simulink library "halin"  (R2021b)
settings: Solver=VariableStepAuto  StartTime=0.0  StopTime=10.0  RelTol=1e-3
undefined symbols (not defined in the file): TRUE
libraries: FVT_lib x177, hcu_lib x55
(part 16 of 17)

== system halin/HAL_IN/CAN4/ZONE_DR_VCU/TFootRErr ==
  T_Foot_R_Err : Inport
  UnitConverter : DataTypeConversion  OutDataTypeStr=uint8
  VHAL_TFootRErr_enum : Outport
  wires:
  UnitConverter/1 -> VHAL_TFootRErr_enum/1
  T_Foot_R_Err/1 -> UnitConverter/1

== system halin/HAL_IN/CAN4/ZONE_DR_VCU/TFootRr ==
  T_Foot_Rr : Inport
  UnitConverter : DataTypeConversion  OutDataTypeStr=uint8
  convert_in : FVT_lib/hal/convert_in  gain=0.5  offset=-40
  VHAL_TFootRr_C : Outport
  wires:
  convert_in/1 -> VHAL_TFootRr_C/1
  UnitConverter/1 -> convert_in/1
  T_Foot_Rr/1 -> UnitConverter/1

== system halin/HAL_IN/CAN4/ZONE_DR_VCU/TFootRrErr ==
  T_Foot_Rr_Err : Inport
  UnitConverter : DataTypeConversion  OutDataTypeStr=uint8
  VHAL_TFootRrErr_enum : Outport
  wires:
  UnitConverter/1 -> VHAL_TFootRrErr_enum/1
  T_Foot_Rr_Err/1 -> UnitConverter/1

== system halin/HAL_IN/CAN4/ZONE_DR_VCU/Tevap ==
  Tevap : Inport
  UnitConverter : DataTypeConversion  OutDataTypeStr=uint8
  convert_in : FVT_lib/hal/convert_in  gain=0.5  offset=-40
  VHAL_Tevap_C : Outport
  wires:
  convert_in/1 -> VHAL_Tevap_C/1
  UnitConverter/1 -> convert_in/1
  Tevap/1 -> UnitConverter/1

== system halin/HAL_IN/CAN4/ZONE_DR_VCU/TevapErr ==
  Tevap_Err : Inport
  UnitConverter : DataTypeConversion  OutDataTypeStr=uint8
  VHAL_TevapErr_enum : Outport
  wires:
  UnitConverter/1 -> VHAL_TevapErr_enum/1
  Tevap_Err/1 -> UnitConverter/1

== system halin/HAL_IN/CAN4/ZONE_DR_VCU/Tincar ==
  Tincar : Inport
  UnitConverter : DataTypeConversion  OutDataTypeStr=uint8
  convert_in : FVT_lib/hal/convert_in  gain=0.5  offset=-40
  VHAL_Tincar_C : Outport
  wires:
  convert_in/1 -> VHAL_Tincar_C/1
  UnitConverter/1 -> convert_in/1
  Tincar/1 -> UnitConverter/1

== system halin/HAL_IN/CAN4/ZONE_DR_VCU/TincarErr ==
  Tincar_Err : Inport
  UnitConverter : DataTypeConversion  OutDataTypeStr=uint8
  VHAL_TincarErr_enum : Outport
  wires:
  UnitConverter/1 -> VHAL_TincarErr_enum/1
  Tincar_Err/1 -> UnitConverter/1

== system halin/HAL_IN/CAN4/ZONE_DR_VCU/ZoneDrMalfunLevel ==
  ZoneDrMalfunLevel : Inport
  UnitConverter : DataTypeConversion  OutDataTypeStr=uint8
  VHAL_ZoneDrMalfunLevel_enum : Outport
  wires:
  UnitConverter/1 -> VHAL_ZoneDrMalfunLevel_enum/1
  ZoneDrMalfunLevel/1 -> UnitConverter/1

== system halin/HAL_IN/CAN4/ZONE_FR1/ChargeInletLockSta ==
  ChargeInletLockSta : Inport
  UnitConverter : DataTypeConversion  OutDataTypeStr=uint8
  VHAL_ChargeInletLockSta_flg : Outport
  wires:
  UnitConverter/1 -> VHAL_ChargeInletLockSta_flg/1
  ChargeInletLockSta/1 -> UnitConverter/1

== system halin/HAL_IN/CAN4/ZONE_FR1/CompProEN ==
  CompProEN : Inport
  UnitConverter : DataTypeConversion  OutDataTypeStr=uint8
  VHAL_CompProEN_flg : Outport
  wires:
  UnitConverter/1 -> VHAL_CompProEN_flg/1
  CompProEN/1 -> UnitConverter/1

== system halin/HAL_IN/CAN4/ZONE_FR1/FLTurnLampC ==
  FLTurnLampC : Inport
  UnitConverter : DataTypeConversion  OutDataTypeStr=uint8
  convert_in : FVT_lib/hal/convert_in  gain=10  offset=0
  VHAL_FLTurnLampC_mA : Outport
  wires:
  convert_in/1 -> VHAL_FLTurnLampC_mA/1
  UnitConverter/1 -> convert_in/1
  FLTurnLampC/1 -> UnitConverter/1

== system halin/HAL_IN/CAN4/ZONE_FR1/FLTurnLightWarning ==
  FLTurn_Light_Warning : Inport
  UnitConverter : DataTypeConversion  OutDataTypeStr=uint8
  VHAL_FLTurnLightWarning_flg : Outport
  wires:
  UnitConverter/1 -> VHAL_FLTurnLightWarning_flg/1
  FLTurn_Light_Warning/1 -> UnitConverter/1

== system halin/HAL_IN/CAN4/ZONE_FR1/FRTurnLampC ==
  FRTurnLampC : Inport
  UnitConverter : DataTypeConversion  OutDataTypeStr=uint8
  convert_in : FVT_lib/hal/convert_in  gain=10  offset=0
  VHAL_FRTurnLampC_mA : Outport
  wires:
  convert_in/1 -> VHAL_FRTurnLampC_mA/1
  UnitConverter/1 -> convert_in/1
  FRTurnLampC/1 -> UnitConverter/1

== system halin/HAL_IN/CAN4/ZONE_FR1/FRTurnLightWarning ==
  FRTurn_Light_Warning : Inport
  UnitConverter : DataTypeConversion  OutDataTypeStr=uint8
  VHAL_FRTurnLightWarning_flg : Outport
  wires:
  UnitConverter/1 -> VHAL_FRTurnLightWarning_flg/1
  FRTurn_Light_Warning/1 -> UnitConverter/1

== system halin/HAL_IN/CAN4/ZONE_FR1/FWiperAS ==
  FWiperAS : Inport
  UnitConverter : DataTypeConversion  OutDataTypeStr=uint8
  VHAL_FWiperAS_flg : Outport
  wires:
  UnitConverter/1 -> VHAL_FWiperAS_flg/1
  FWiperAS/1 -> UnitConverter/1

== system halin/HAL_IN/CAN4/ZONE_FR1/FWiperProtection ==
  FWiperProtection : Inport
  UnitConverter : DataTypeConversion  OutDataTypeStr=uint8
  VHAL_FWiperProtection_flg : Outport
  wires:
  UnitConverter/1 -> VHAL_FWiperProtection_flg/1
  FWiperProtection/1 -> UnitConverter/1

== system halin/HAL_IN/CAN4/ZONE_FR1/LADBHibeamIndication ==
  LADB_Hibeam_Indication : Inport
  UnitConverter : DataTypeConversion  OutDataTypeStr=uint8
  VHAL_LADBHibeamIndication_flg : Outport
  wires:
  UnitConverter/1 -> VHAL_LADBHibeamIndication_flg/1
  LADB_Hibeam_Indication/1 -> UnitConverter/1

== system halin/HAL_IN/CAN4/ZONE_FR1/LADBOperationStatus ==
  LADB_Operation_Status : Inport
  UnitConverter : DataTypeConversion  OutDataTypeStr=uint8
  VHAL_LADBOperationStatus_flg : Outport
  wires:
  UnitConverter/1 -> VHAL_LADBOperationStatus_flg/1
  LADB_Operation_Status/1 -> UnitConverter/1

== system halin/HAL_IN/CAN4/ZONE_FR1/LADBWarning ==
  LADB_Warning : Inport
  UnitConverter : DataTypeConversion  OutDataTypeStr=uint8
  VHAL_LADBWarning_flg : Outport
  wires:
  UnitConverter/1 -> VHAL_LADBWarning_flg/1
  LADB_Warning/1 -> UnitConverter/1

== system halin/HAL_IN/CAN4/ZONE_FR1/LAHBWarning ==
  LAHB_Warning : Inport
  UnitConverter : DataTypeConversion  OutDataTypeStr=uint8
  VHAL_LAHBWarning_flg : Outport
  wires:
  UnitConverter/1 -> VHAL_LAHBWarning_flg/1
  LAHB_Warning/1 -> UnitConverter/1

== system halin/HAL_IN/CAN4/ZONE_FR1/LDRLWarning ==
  LDRL_Warning : Inport
  UnitConverter : DataTypeConversion  OutDataTypeStr=uint8
  VHAL_LDRLWarning_flg : Outport
  wires:
  UnitConverter/1 -> VHAL_LDRLWarning_flg/1
  LDRL_Warning/1 -> UnitConverter/1

== system halin/HAL_IN/CAN4/ZONE_FR1/LLBWarning ==
  LLB_Warning : Inport
  UnitConverter : DataTypeConversion  OutDataTypeStr=uint8
  VHAL_LLBWarning_flg : Outport
  wires:
  UnitConverter/1 -> VHAL_LLBWarning_flg/1
  LLB_Warning/1 -> UnitConverter/1

== system halin/HAL_IN/CAN4/ZONE_FR1/LpositionLampWarning ==
  Lposition_Lamp_Warning : Inport
  UnitConverter : DataTypeConversion  OutDataTypeStr=uint8
  VHAL_LpositionLampWarning_flg : Outport
  wires:
  UnitConverter/1 -> VHAL_LpositionLampWarning_flg/1
  Lposition_Lamp_Warning/1 -> UnitConverter/1

== system halin/HAL_IN/CAN4/ZONE_FR1/RADBHibeamIndication ==
  RADB_Hibeam_Indication : Inport
  UnitConverter : DataTypeConversion  OutDataTypeStr=uint8
  VHAL_RADBHibeamIndication_flg : Outport
  wires:
  UnitConverter/1 -> VHAL_RADBHibeamIndication_flg/1
  RADB_Hibeam_Indication/1 -> UnitConverter/1

== system halin/HAL_IN/CAN4/ZONE_FR1/RADBOperationStatus ==
  RADB_Operation_Status : Inport
  UnitConverter : DataTypeConversion  OutDataTypeStr=uint8
  VHAL_RADBOperationStatus_flg : Outport
  wires:
  UnitConverter/1 -> VHAL_RADBOperationStatus_flg/1
  RADB_Operation_Status/1 -> UnitConverter/1

== system halin/HAL_IN/CAN4/ZONE_FR1/RADBWarning ==
  RADB_Warning : Inport
  UnitConverter : DataTypeConversion  OutDataTypeStr=uint8
  VHAL_RADBWarning_flg : Outport
  wires:
  UnitConverter/1 -> VHAL_RADBWarning_flg/1
  RADB_Warning/1 -> UnitConverter/1

== system halin/HAL_IN/CAN4/ZONE_FR1/RAHBWarning ==
  RAHB_Warning : Inport
  UnitConverter : DataTypeConversion  OutDataTypeStr=uint8
  VHAL_RAHBWarning_flg : Outport
  wires:
  UnitConverter/1 -> VHAL_RAHBWarning_flg/1
  RAHB_Warning/1 -> UnitConverter/1

== system halin/HAL_IN/CAN4/ZONE_FR1/RDRLWarning ==
  RDRL_Warning : Inport
  UnitConverter : DataTypeConversion  OutDataTypeStr=uint8
  VHAL_RDRLWarning_flg : Outport
  wires:
  UnitConverter/1 -> VHAL_RDRLWarning_flg/1
  RDRL_Warning/1 -> UnitConverter/1

== system halin/HAL_IN/CAN4/ZONE_FR1/RLBWarning ==
  RLB_Warning : Inport
  UnitConverter : DataTypeConversion  OutDataTypeStr=uint8
  VHAL_RLBWarning_flg : Outport
  wires:
  UnitConverter/1 -> VHAL_RLBWarning_flg/1
  RLB_Warning/1 -> UnitConverter/1

== system halin/HAL_IN/CAN4/ZONE_FR1/RpositionLampWarning ==
  Rposition_Lamp_Warning : Inport
  UnitConverter : DataTypeConversion  OutDataTypeStr=uint8
  VHAL_RpositionLampWarning_flg : Outport
  wires:
  UnitConverter/1 -> VHAL_RpositionLampWarning_flg/1
  Rposition_Lamp_Warning/1 -> UnitConverter/1

== system halin/HAL_IN/CAN4/ZONE_FR1/TrailerCheck ==
  TrailerCheck : Inport
  UnitConverter : DataTypeConversion  OutDataTypeStr=uint8
  VHAL_TrailerCheck_flg : Outport
  wires:
  UnitConverter/1 -> VHAL_TrailerCheck_flg/1
  TrailerCheck/1 -> UnitConverter/1

== system halin/HAL_IN/CAN4/ZONE_FR1/TrailerModeSta ==
  TrailerModeSta : Inport
  UnitConverter : DataTypeConversion  OutDataTypeStr=uint8
  VHAL_TrailerModeSta_enum : Outport
  wires:
  UnitConverter/1 -> VHAL_TrailerModeSta_enum/1
  TrailerModeSta/1 -> UnitConverter/1

== system halin/HAL_IN/CAN4/ZONE_FR1/ZFRBCMChargerDoorSWSta ==
  ZFR_BCM_ChargerDoorSW_Sta : Inport
  UnitConverter : DataTypeConversion  OutDataTypeStr=uint8
  VHAL_ZFRBCMChargerDoorSWSta_flg : Outport
  wires:
  UnitConverter/1 -> VHAL_ZFRBCMChargerDoorSWSta_flg/1
  ZFR_BCM_ChargerDoorSW_Sta/1 -> UnitConverter/1

== system halin/HAL_IN/CAN4/ZONE_FR1/ZFRTHCMCLEVentActYSta ==
  ZFR_THCM_CLEVentActY_Sta : Inport
  UnitConverter : DataTypeConversion  OutDataTypeStr=uint8
  VHAL_ZFRTHCMCLEVentActYSta_pct : Outport
  wires:
  UnitConverter/1 -> VHAL_ZFRTHCMCLEVentActYSta_pct/1
  ZFR_THCM_CLEVentActY_Sta/1 -> UnitConverter/1

== system halin/HAL_IN/CAN4/ZONE_FR1/ZFRTHCMCREVentActYSta ==
  ZFR_THCM_CREVentActY_Sta : Inport
  UnitConverter : DataTypeConversion  OutDataTypeStr=uint8
  VHAL_ZFRTHCMCREVentActYSta_pct : Outport
  wires:
  UnitConverter/1 -> VHAL_ZFRTHCMCREVentActYSta_pct/1
  ZFR_THCM_CREVentActY_Sta/1 -> UnitConverter/1

== system halin/HAL_IN/CAN4/ZONE_FR1/ZFRTHCMDrEVentActYSta ==
  ZFR_THCM_DrEVentActY_Sta : Inport
  UnitConverter : DataTypeConversion  OutDataTypeStr=uint8
  VHAL_ZFRTHCMDrEVentActYSta_pct : Outport
  wires:
  UnitConverter/1 -> VHAL_ZFRTHCMDrEVentActYSta_pct/1
  ZFR_THCM_DrEVentActY_Sta/1 -> UnitConverter/1

== system halin/HAL_IN/CAN4/ZONE_FR1/ZFRTHCMPsEVentActYSta ==
  ZFR_THCM_PsEVentActY_Sta : Inport
  UnitConverter : DataTypeConversion  OutDataTypeStr=uint8
  VHAL_ZFRTHCMPsEVentActYSta_pct : Outport
  wires:
  UnitConverter/1 -> VHAL_ZFRTHCMPsEVentActYSta_pct/1
  ZFR_THCM_PsEVentActY_Sta/1 -> UnitConverter/1

== system halin/HAL_IN/CAN4/ZONE_FR_VCU/AGSErr ==
  AGS_Err : Inport
  UnitConverter : DataTypeConversion  OutDataTypeStr=uint8
  VHAL_AGSErr_enum : Outport
  wires:
  UnitConverter/1 -> VHAL_AGSErr_enum/1
  AGS_Err/1 -> UnitConverter/1

== system halin/HAL_IN/CAN4/ZONE_FR_VCU/BatInTemp ==
  Bat_In_Temp : Inport
  UnitConverter : DataTypeConversion  OutDataTypeStr=uint8
  convert_in : FVT_lib/hal/convert_in  gain=0.5  offset=-40
  VHAL_BatInTemp_C : Outport
  wires:
  convert_in/1 -> VHAL_BatInTemp_C/1
  UnitConverter/1 -> convert_in/1
  Bat_In_Temp/1 -> UnitConverter/1

== system halin/HAL_IN/CAN4/ZONE_FR_VCU/BatInTempErr ==
  Bat_In_Temp_Err : Inport
  UnitConverter : DataTypeConversion  OutDataTypeStr=uint8
  VHAL_BatInTempErr_enum : Outport
  wires:
  UnitConverter/1 -> VHAL_BatInTempErr_enum/1
  Bat_In_Temp_Err/1 -> UnitConverter/1

== system halin/HAL_IN/CAN4/ZONE_FR_VCU/BatOutTemp ==
  Bat_Out_Temp : Inport
  UnitConverter : DataTypeConversion  OutDataTypeStr=uint8
  convert_in : FVT_lib/hal/convert_in  gain=0.5  offset=-40
  VHAL_BatOutTemp_C : Outport
  wires:
  convert_in/1 -> VHAL_BatOutTemp_C/1
  UnitConverter/1 -> convert_in/1
  Bat_Out_Temp/1 -> UnitConverter/1

== system halin/HAL_IN/CAN4/ZONE_FR_VCU/COMPErr ==
  COMP_Err : Inport
  UnitConverter : DataTypeConversion  OutDataTypeStr=uint8
  VHAL_COMPErr_enum : Outport
  wires:
  UnitConverter/1 -> VHAL_COMPErr_enum/1
  COMP_Err/1 -> UnitConverter/1

== system halin/HAL_IN/CAN4/ZONE_FR_VCU/EACProtectEnable ==
  EACProtectEnable : Inport
  UnitConverter : DataTypeConversion  OutDataTypeStr=uint8
  VHAL_EACProtectEnable_enum : Outport
  wires:
  UnitConverter/1 -> VHAL_EACProtectEnable_enum/1
  EACProtectEnable/1 -> UnitConverter/1

== system halin/HAL_IN/CAN4/ZONE_FR_VCU/EWP3Err ==
  EWP3_Err : Inport
  UnitConverter : DataTypeConversion  OutDataTypeStr=uint8
  VHAL_EWP3Err_enum : Outport
  wires:
  UnitConverter/1 -> VHAL_EWP3Err_enum/1
  EWP3_Err/1 -> UnitConverter/1

== system halin/HAL_IN/CAN4/ZONE_FR_VCU/EXV1Err ==
  EXV1_Err : Inport
  UnitConverter : DataTypeConversion  OutDataTypeStr=uint8
  VHAL_EXV1Err_enum : Outport
  wires:
  UnitConverter/1 -> VHAL_EXV1Err_enum/1
  EXV1_Err/1 -> UnitConverter/1

== system halin/HAL_IN/CAN4/ZONE_FR_VCU/EXV2Err ==
  EXV2_Err : Inport
  UnitConverter : DataTypeConversion  OutDataTypeStr=uint8
  VHAL_EXV2Err_enum : Outport
  wires:
  UnitConverter/1 -> VHAL_EXV2Err_enum/1
  EXV2_Err/1 -> UnitConverter/1

== system halin/HAL_IN/CAN4/ZONE_FR_VCU/FanErr ==
  Fan_Err : Inport
  UnitConverter : DataTypeConversion  OutDataTypeStr=uint8
  VHAL_FanErr_enum : Outport
  wires:
  UnitConverter/1 -> VHAL_FanErr_enum/1
  Fan_Err/1 -> UnitConverter/1

== system halin/HAL_IN/CAN4/ZONE_FR_VCU/FrPMMLimpHomeActReq ==
  FrPMMLimpHomeActReq : Inport
  UnitConverter : DataTypeConversion  OutDataTypeStr=uint8
  VHAL_FrPMMLimpHomeActReq_flg : Outport
  wires:
  UnitConverter/1 -> VHAL_FrPMMLimpHomeActReq_flg/1
  FrPMMLimpHomeActReq/1 -> UnitConverter/1

== system halin/HAL_IN/CAN4/ZONE_FR_VCU/MotorInTemp ==
  Motor_In_Temp : Inport
  UnitConverter : DataTypeConversion  OutDataTypeStr=uint8
  convert_in : FVT_lib/hal/convert_in  gain=0.5  offset=-40
  VHAL_MotorInTemp_C : Outport
  wires:
  convert_in/1 -> VHAL_MotorInTemp_C/1
  UnitConverter/1 -> convert_in/1
  Motor_In_Temp/1 -> UnitConverter/1

== system halin/HAL_IN/CAN4/ZONE_FR_VCU/MotorInTempErr ==
  Motor_In_Temp_Err : Inport
  UnitConverter : DataTypeConversion  OutDataTypeStr=uint8
  VHAL_MotorInTempErr_enum : Outport
  wires:
  UnitConverter/1 -> VHAL_MotorInTempErr_enum/1
  Motor_In_Temp_Err/1 -> UnitConverter/1

== system halin/HAL_IN/CAN4/ZONE_FR_VCU/MotorOutTemp ==
  Motor_Out_Temp : Inport
  UnitConverter : DataTypeConversion  OutDataTypeStr=uint8
  convert_in : FVT_lib/hal/convert_in  gain=0.5  offset=-40
  VHAL_MotorOutTemp_C : Outport
  wires:
  convert_in/1 -> VHAL_MotorOutTemp_C/1
  UnitConverter/1 -> convert_in/1
  Motor_Out_Temp/1 -> UnitConverter/1

== system halin/HAL_IN/CAN4/ZONE_FR_VCU/MotorOutTempErr ==
  Motor_Out_Temp_Err : Inport
  UnitConverter : DataTypeConversion  OutDataTypeStr=uint8
  VHAL_MotorOutTempErr_enum : Outport
  wires:
  UnitConverter/1 -> VHAL_MotorOutTempErr_enum/1
  Motor_Out_Temp_Err/1 -> UnitConverter/1

== system halin/HAL_IN/CAN4/ZONE_FR_VCU/PTHighP ==
  PT_High_P : Inport
  UnitConverter : DataTypeConversion  OutDataTypeStr=uint16
  VHAL_PTHighP_KPa : Outport
  wires:
  UnitConverter/1 -> VHAL_PTHighP_KPa/1
  PT_High_P/1 -> UnitConverter/1

== system halin/HAL_IN/CAN4/ZONE_FR_VCU/PTHighPErr ==
  PT_High_P_Err : Inport
  UnitConverter : DataTypeConversion  OutDataTypeStr=uint8
  VHAL_PTHighPErr_enum : Outport
  wires:
  UnitConverter/1 -> VHAL_PTHighPErr_enum/1
  PT_High_P_Err/1 -> UnitConverter/1

== system halin/HAL_IN/CAN4/ZONE_FR_VCU/PTHighTact ==
  PT_High_Tact : Inport
  UnitConverter : DataTypeConversion  OutDataTypeStr=uint8
  convert_in : FVT_lib/hal/convert_in  gain=1  offset=-40
  VHAL_PTHighTact_C : Outport
  wires:
  convert_in/1 -> VHAL_PTHighTact_C/1
  UnitConverter/1 -> convert_in/1
  PT_High_Tact/1 -> UnitConverter/1

== system halin/HAL_IN/CAN4/ZONE_FR_VCU/PTHighTactErr ==
  PT_High_Tact_Err : Inport
  UnitConverter : DataTypeConversion  OutDataTypeStr=uint8
  VHAL_PTHighTactErr_enum : Outport
  wires:
  UnitConverter/1 -> VHAL_PTHighTactErr_enum/1
  PT_High_Tact_Err/1 -> UnitConverter/1

== system halin/HAL_IN/CAN4/ZONE_FR_VCU/PTLowP1 ==
  PT_Low_P1 : Inport
  UnitConverter : DataTypeConversion  OutDataTypeStr=uint16
  VHAL_PTLowP1_KPa : Outport
  wires:
  UnitConverter/1 -> VHAL_PTLowP1_KPa/1
  PT_Low_P1/1 -> UnitConverter/1

== system halin/HAL_IN/CAN4/ZONE_FR_VCU/PTLowP1Err ==
  PT_Low_P1_Err : Inport
  UnitConverter : DataTypeConversion  OutDataTypeStr=uint8
  VHAL_PTLowP1Err_enum : Outport
  wires:
  UnitConverter/1 -> VHAL_PTLowP1Err_enum/1
  PT_Low_P1_Err/1 -> UnitConverter/1

== system halin/HAL_IN/CAN4/ZONE_FR_VCU/PTLowP2 ==
  PT_Low_P2 : Inport
  UnitConverter : DataTypeConversion  OutDataTypeStr=uint16
  VHAL_PTLowP2_KPa : Outport
  wires:
  UnitConverter/1 -> VHAL_PTLowP2_KPa/1
  PT_Low_P2/1 -> UnitConverter/1

== system halin/HAL_IN/CAN4/ZONE_FR_VCU/PTLowP2Err ==
  PT_Low_P2_Err : Inport
  UnitConverter : DataTypeConversion  OutDataTypeStr=uint8
  VHAL_PTLowP2Err_enum : Outport
  wires:
  UnitConverter/1 -> VHAL_PTLowP2Err_enum/1
  PT_Low_P2_Err/1 -> UnitConverter/1

== system halin/HAL_IN/CAN4/ZONE_FR_VCU/PTLowT1 ==
  PT_Low_T1 : Inport
  UnitConverter : DataTypeConversion  OutDataTypeStr=uint8
  convert_in : FVT_lib/hal/convert_in  gain=0.5  offset=-40
  VHAL_PTLowT1_C : Outport
  wires:
  convert_in/1 -> VHAL_PTLowT1_C/1
  UnitConverter/1 -> convert_in/1
  PT_Low_T1/1 -> UnitConverter/1

== system halin/HAL_IN/CAN4/ZONE_FR_VCU/PTLowT1Err ==
  PT_Low_T1_Err : Inport
  UnitConverter : DataTypeConversion  OutDataTypeStr=uint8
  VHAL_PTLowT1Err_enum : Outport
  wires:
  UnitConverter/1 -> VHAL_PTLowT1Err_enum/1
  PT_Low_T1_Err/1 -> UnitConverter/1

== system halin/HAL_IN/CAN4/ZONE_FR_VCU/PTLowT2 ==
  PT_Low_T2 : Inport
  UnitConverter : DataTypeConversion  OutDataTypeStr=uint8
  convert_in : FVT_lib/hal/convert_in  gain=0.5  offset=-40
  VHAL_PTLowT2_C : Outport
  wires:
  convert_in/1 -> VHAL_PTLowT2_C/1
  UnitConverter/1 -> convert_in/1
  PT_Low_T2/1 -> UnitConverter/1

== system halin/HAL_IN/CAN4/ZONE_FR_VCU/PTLowT2Err ==
  PT_Low_T2_Err : Inport
  UnitConverter : DataTypeConversion  OutDataTypeStr=uint8
  VHAL_PTLowT2Err_enum : Outport
  wires:
  UnitConverter/1 -> VHAL_PTLowT2Err_enum/1
  PT_Low_T2_Err/1 -> UnitConverter/1

== system halin/HAL_IN/CAN4/ZONE_FR_VCU/SOTXVErr ==
  SOTXV_Err : Inport
  UnitConverter : DataTypeConversion  OutDataTypeStr=uint8
  VHAL_SOTXVErr_enum : Outport
  wires:
  UnitConverter/1 -> VHAL_SOTXVErr_enum/1
  SOTXV_Err/1 -> UnitConverter/1

== system halin/HAL_IN/CAN4/ZONE_FR_VCU/SOV1Err ==
  SOV1_Err : Inport
  UnitConverter : DataTypeConversion  OutDataTypeStr=uint8
  VHAL_SOV1Err_enum : Outport
  wires:
  UnitConverter/1 -> VHAL_SOV1Err_enum/1
  SOV1_Err/1 -> UnitConverter/1

== system halin/HAL_IN/CAN4/ZONE_FR_VCU/SOV2Err ==
  SOV2_Err : Inport
  UnitConverter : DataTypeConversion  OutDataTypeStr=uint8
  VHAL_SOV2Err_enum : Outport
  wires:
  UnitConverter/1 -> VHAL_SOV2Err_enum/1
  SOV2_Err/1 -> UnitConverter/1

== system halin/HAL_IN/CAN4/ZONE_FR_VCU/SOV3Err ==
  SOV3_Err : Inport
  UnitConverter : DataTypeConversion  OutDataTypeStr=uint8
  VHAL_SOV3Err_enum : Outport
  wires:
  UnitConverter/1 -> VHAL_SOV3Err_enum/1
  SOV3_Err/1 -> UnitConverter/1

== system halin/HAL_IN/CAN4/ZONE_FR_VCU/Tamb ==
  Tamb : Inport
  UnitConverter : DataTypeConversion  OutDataTypeStr=uint8
  convert_in : FVT_lib/hal/convert_in  gain=0.5  offset=-40
  VHAL_Tamb_C : Outport
  wires:
  convert_in/1 -> VHAL_Tamb_C/1
  UnitConverter/1 -> convert_in/1
  Tamb/1 -> UnitConverter/1

== system halin/HAL_IN/CAN4/ZONE_FR_VCU/TambErr ==
  Tamb_Err : Inport
  UnitConverter : DataTypeConversion  OutDataTypeStr=uint8
  VHAL_TambErr_enum : Outport
  wires:
  UnitConverter/1 -> VHAL_TambErr_enum/1
  Tamb_Err/1 -> UnitConverter/1

== system halin/HAL_IN/CAN4/ZONE_L1/ZLDSEATAntiSta ==
  ZL_DSEAT_Anti_Sta : Inport
  UnitConverter : DataTypeConversion  OutDataTypeStr=uint8
  VHAL_ZLDSEATAntiSta_flg : Outport
  wires:
  UnitConverter/1 -> VHAL_ZLDSEATAntiSta_flg/1
  ZL_DSEAT_Anti_Sta/1 -> UnitConverter/1

== system halin/HAL_IN/CAN4/ZONE_L1/ZLDSEATEntryFunSta ==
  ZL_DSEAT_EntryFun_Sta : Inport
  UnitConverter : DataTypeConversion  OutDataTypeStr=uint8
  VHAL_ZLDSEATEntryFunSta_flg : Outport
  wires:
  UnitConverter/1 -> VHAL_ZLDSEATEntryFunSta_flg/1
  ZL_DSEAT_EntryFun_Sta/1 -> UnitConverter/1

== system halin/HAL_IN/CAN4/ZONE_L1/ZLDSEATErrorSta ==
  ZL_DSEAT_Error_Sta : Inport
  UnitConverter : DataTypeConversion  OutDataTypeStr=uint8
  VHAL_ZLDSEATErrorSta_flg : Outport
  wires:
  UnitConverter/1 -> VHAL_ZLDSEATErrorSta_flg/1
  ZL_DSEAT_Error_Sta/1 -> UnitConverter/1

== system halin/HAL_IN/CAN4/ZONE_L1/ZLDSEATMemSetSta ==
  ZL_DSEAT_MemSet_Sta : Inport
  UnitConverter : DataTypeConversion  OutDataTypeStr=uint8
  VHAL_ZLDSEATMemSetSta_enum : Outport
  wires:
  UnitConverter/1 -> VHAL_ZLDSEATMemSetSta_enum/1
  ZL_DSEAT_MemSet_Sta/1 -> UnitConverter/1

== system halin/HAL_IN/CAN4/ZONE_L1/ZLDSEATModeSta ==
  ZL_DSEAT_Mode_Sta : Inport
  UnitConverter : DataTypeConversion  OutDataTypeStr=uint8
  VHAL_ZLDSEATModeSta_enum : Outport
  wires:
  UnitConverter/1 -> VHAL_ZLDSEATModeSta_enum/1
  ZL_DSEAT_Mode_Sta/1 -> UnitConverter/1

== system halin/HAL_IN/CAN4/ZONE_L1/ZLDSEATVentSta ==
  ZL_DSEAT_Vent_Sta : Inport
  UnitConverter : DataTypeConversion  OutDataTypeStr=uint8
  VHAL_ZLDSEATVentSta_enum : Outport
  wires:
  UnitConverter/1 -> VHAL_ZLDSEATVentSta_enum/1
  ZL_DSEAT_Vent_Sta/1 -> UnitConverter/1

== system halin/HAL_IN/CAN4/ZONE_L1/ZLDSEATheaterSta ==
  ZL_DSEAT_heater_Sta : Inport
  UnitConverter : DataTypeConversion  OutDataTypeStr=uint8
  VHAL_ZLDSEATheaterSta_enum : Outport
  wires:
  UnitConverter/1 -> VHAL_ZLDSEATheaterSta_enum/1
  ZL_DSEAT_heater_Sta/1 -> UnitConverter/1

== system halin/HAL_IN/CAN4/ZONE_L2/ZLAPMWinLFOpenedSta ==
  ZL_APM_WinLFOpened_Sta : Inport
  UnitConverter : DataTypeConversion  OutDataTypeStr=uint8
  VHAL_ZLAPMWinLFOpenedSta_pct : Outport
  wires:
  UnitConverter/1 -> VHAL_ZLAPMWinLFOpenedSta_pct/1
  ZL_APM_WinLFOpened_Sta/1 -> UnitConverter/1

== system halin/HAL_IN/CAN4/ZONE_L2/ZLAPMWinLROpenedSta ==
  ZL_APM_WinLROpened_Sta : Inport
  UnitConverter : DataTypeConversion  OutDataTypeStr=uint8
  VHAL_ZLAPMWinLROpenedSta_pct : Outport
  wires:
  UnitConverter/1 -> VHAL_ZLAPMWinLROpenedSta_pct/1
  ZL_APM_WinLROpened_Sta/1 -> UnitConverter/1

== system halin/HAL_IN/CAN4/ZONE_R1/ZRPSEATErrorSta ==
  ZR_PSEAT_Error_Sta : Inport
  UnitConverter : DataTypeConversion  OutDataTypeStr=uint8
  VHAL_ZRPSEATErrorSta_flg : Outport
  wires:
  UnitConverter/1 -> VHAL_ZRPSEATErrorSta_flg/1
  ZR_PSEAT_Error_Sta/1 -> UnitConverter/1

== system halin/HAL_IN/CAN4/ZONE_R1/ZRPSEATModeSta ==
  ZR_PSEAT_Mode_Sta : Inport
  UnitConverter : DataTypeConversion  OutDataTypeStr=uint8
  VHAL_ZRPSEATModeSta_enum : Outport
  wires:
  UnitConverter/1 -> VHAL_ZRPSEATModeSta_enum/1
  ZR_PSEAT_Mode_Sta/1 -> UnitConverter/1

== system halin/HAL_IN/CAN4/ZONE_R1/ZRPSEATVentSta ==
  ZR_PSEAT_Vent_Sta : Inport
  UnitConverter : DataTypeConversion  OutDataTypeStr=uint8
  VHAL_ZRPSEATVentSta_enum : Outport
  wires:
  UnitConverter/1 -> VHAL_ZRPSEATVentSta_enum/1
  ZR_PSEAT_Vent_Sta/1 -> UnitConverter/1

== system halin/HAL_IN/CAN4/ZONE_R1/ZRPSEATheaterSta ==
  ZR_PSEAT_heater_Sta : Inport
  UnitConverter : DataTypeConversion  OutDataTypeStr=uint8
  VHAL_ZRPSEATheaterSta_enum : Outport
  wires:
  UnitConverter/1 -> VHAL_ZRPSEATheaterSta_enum/1
  ZR_PSEAT_heater_Sta/1 -> UnitConverter/1

== system halin/HAL_IN/CAN4/ZONE_R1/ZRPTGActiveSta ==
  ZR_PTG_Active_Sta : Inport
  UnitConverter : DataTypeConversion  OutDataTypeStr=uint8
  VHAL_ZRPTGActiveSta_enum : Outport
  wires:
  UnitConverter/1 -> VHAL_ZRPTGActiveSta_enum/1
  ZR_PTG_Active_Sta/1 -> UnitConverter/1

== system halin/HAL_IN/CAN4/ZONE_R1/ZRPTGExistSta ==
  ZR_PTG_Exist_Sta : Inport
  UnitConverter : DataTypeConversion  OutDataTypeStr=uint8
  VHAL_ZRPTGExistSta_flg : Outport
  wires:
  UnitConverter/1 -> VHAL_ZRPTGExistSta_flg/1
  ZR_PTG_Exist_Sta/1 -> UnitConverter/1

== system halin/HAL_IN/CAN4/ZONE_R1/ZRPTGIsSetHeightSta ==
  ZR_PTG_IsSetHeight_Sta : Inport
  UnitConverter : DataTypeConversion  OutDataTypeStr=uint8
  VHAL_ZRPTGIsSetHeightSta_flg : Outport
  wires:
  UnitConverter/1 -> VHAL_ZRPTGIsSetHeightSta_flg/1
  ZR_PTG_IsSetHeight_Sta/1 -> UnitConverter/1

== system halin/HAL_IN/CAN4/ZONE_R1/ZRPTGSysSta ==
  ZR_PTG_Sys_Sta : Inport
  UnitConverter : DataTypeConversion  OutDataTypeStr=uint8
  VHAL_ZRPTGSysSta_enum : Outport
  wires:
  UnitConverter/1 -> VHAL_ZRPTGSysSta_enum/1
  ZR_PTG_Sys_Sta/1 -> UnitConverter/1

== system halin/HAL_IN/CAN4/ZONE_R2/ZRAPMWinRFOpenedSta ==
  ZR_APM_WinRFOpened_Sta : Inport
  UnitConverter : DataTypeConversion  OutDataTypeStr=uint8
  VHAL_ZRAPMWinRFOpenedSta_pct : Outport
  wires:
  UnitConverter/1 -> VHAL_ZRAPMWinRFOpenedSta_pct/1
  ZR_APM_WinRFOpened_Sta/1 -> UnitConverter/1

== system halin/HAL_IN/CAN4/ZONE_R2/ZRAPMWinRROpenedSta ==
  ZR_APM_WinRROpened_Sta : Inport
  UnitConverter : DataTypeConversion  OutDataTypeStr=uint8
  VHAL_ZRAPMWinRROpenedSta_pct : Outport
  wires:
  UnitConverter/1 -> VHAL_ZRAPMWinRROpenedSta_pct/1
  ZR_APM_WinRROpened_Sta/1 -> UnitConverter/1

== system halin/HAL_IN/CAN4/ZONE_R2/ZRSEATLVentSta ==
  ZR_SEAT_LVent_Sta : Inport
  UnitConverter : DataTypeConversion  OutDataTypeStr=uint8
  VHAL_ZRSEATLVentSta_enum : Outport
  wires:
  UnitConverter/1 -> VHAL_ZRSEATLVentSta_enum/1
  ZR_SEAT_LVent_Sta/1 -> UnitConverter/1

== system halin/HAL_IN/CAN4/ZONE_R2/ZRSEATMLVentSta ==
  ZR_SEAT_MLVent_Sta : Inport
  UnitConverter : DataTypeConversion  OutDataTypeStr=uint8
  VHAL_ZRSEATMLVentSta_enum : Outport
  wires:
  UnitConverter/1 -> VHAL_ZRSEATMLVentSta_enum/1
  ZR_SEAT_MLVent_Sta/1 -> UnitConverter/1

== system halin/HAL_IN/CAN4/ZONE_R2/ZRSEATMRVentSta ==
  ZR_SEAT_MRVent_Sta : Inport
  UnitConverter : DataTypeConversion  OutDataTypeStr=uint8
  VHAL_ZRSEATMRVentSta_enum : Outport
  wires:
  UnitConverter/1 -> VHAL_ZRSEATMRVentSta_enum/1
  ZR_SEAT_MRVent_Sta/1 -> UnitConverter/1

== system halin/HAL_IN/CAN4/ZONE_R2/ZRSEATRVentSta ==
  ZR_SEAT_RVent_Sta : Inport
  UnitConverter : DataTypeConversion  OutDataTypeStr=uint8
  VHAL_ZRSEATRVentSta_enum : Outport
  wires:
  UnitConverter/1 -> VHAL_ZRSEATRVentSta_enum/1
  ZR_SEAT_RVent_Sta/1 -> UnitConverter/1

== system halin/HAL_IN/CAN4/zGW_APTC1/FrntPTCLeActHeatPwr ==
  FrntPTCLeActHeatPwr : Inport
  UnitConverter : DataTypeConversion  OutDataTypeStr=uint8
  convert_in : FVT_lib/hal/convert_in  gain=25  offset=0
  VHAL_FrntPTCLeActHeatPwr_W : Outport
  wires:
  convert_in/1 -> VHAL_FrntPTCLeActHeatPwr_W/1
  UnitConverter/1 -> convert_in/1
  FrntPTCLeActHeatPwr/1 -> UnitConverter/1

== system halin/HAL_IN/CAN4/zGW_APTC1/FrntPTCRearLeActHeatPwr ==
  FrntPTCRearLeActHeatPwr : Inport
  UnitConverter : DataTypeConversion  OutDataTypeStr=uint8
  convert_in : FVT_lib/hal/convert_in  gain=25  offset=0
  VHAL_FrntPTCRearLeActHeatPwr_W : Outport
  wires:
  convert_in/1 -> VHAL_FrntPTCRearLeActHeatPwr_W/1
  UnitConverter/1 -> convert_in/1
  FrntPTCRearLeActHeatPwr/1 -> UnitConverter/1

== system halin/HAL_IN/CAN4/zGW_APTC1/FrntPTCRearRiActHeatPwr ==
  FrntPTCRearRiActHeatPwr : Inport
  UnitConverter : DataTypeConversion  OutDataTypeStr=uint8
  convert_in : FVT_lib/hal/convert_in  gain=25  offset=0
  VHAL_FrntPTCRearRiActHeatPwr_W : Outport
  wires:
  convert_in/1 -> VHAL_FrntPTCRearRiActHeatPwr_W/1
  UnitConverter/1 -> convert_in/1
  FrntPTCRearRiActHeatPwr/1 -> UnitConverter/1

== system halin/HAL_IN/CAN4/zGW_APTC1/FrntPTCRiActHeatPwr ==
  FrntPTCRiActHeatPwr : Inport
  UnitConverter : DataTypeConversion  OutDataTypeStr=uint8
  convert_in : FVT_lib/hal/convert_in  gain=25  offset=0
  VHAL_FrntPTCRiActHeatPwr_W : Outport
  wires:
  convert_in/1 -> VHAL_FrntPTCRiActHeatPwr_W/1
  UnitConverter/1 -> convert_in/1
  FrntPTCRiActHeatPwr/1 -> UnitConverter/1

== system halin/HAL_IN/CAN4/zGW_CANFr1/COMPActualPwr ==
  COMP_ActualPwr : Inport
  UnitConverter : DataTypeConversion  OutDataTypeStr=uint16
  VHAL_COMPActualPwr_W : Outport
  wires:
  UnitConverter/1 -> VHAL_COMPActualPwr_W/1
  COMP_ActualPwr/1 -> UnitConverter/1

== system halin/HAL_IN/CAN4/zGW_CANFr1/COMPConCur ==
  COMP_ConCur : Inport
  UnitConverter : DataTypeConversion  OutDataTypeStr=uint16
  convert_in : FVT_lib/hal/convert_in  gain=0.02  offset=0
  VHAL_COMPConCur_A : Outport
  wires:
  convert_in/1 -> VHAL_COMPConCur_A/1
  UnitConverter/1 -> convert_in/1
  COMP_ConCur/1 -> UnitConverter/1

== system halin/HAL_IN/CAN4/zGW_CANFr1/COMPConVolt ==
  COMP_ConVolt : Inport
  UnitConverter : DataTypeConversion  OutDataTypeStr=uint16
  convert_in : FVT_lib/hal/convert_in  gain=0.02  offset=0
  VHAL_COMPConVolt_V : Outport
  wires:
  convert_in/1 -> VHAL_COMPConVolt_V/1
  UnitConverter/1 -> convert_in/1
  COMP_ConVolt/1 -> UnitConverter/1

== system halin/HAL_IN/CAN4/zGW_CANFr1/COMPStatorSpd ==
  COMP_StatorSpd : Inport
  UnitConverter : DataTypeConversion  OutDataTypeStr=uint16
  VHAL_COMPStatorSpd_rpm : Outport
  wires:
  UnitConverter/1 -> VHAL_COMPStatorSpd_rpm/1
  COMP_StatorSpd/1 -> UnitConverter/1

== system halin/HAL_IN/CAN4/zGW_CANFr1/PTC1PowerConsumption ==
  PTC1_PowerConsumption : Inport
  UnitConverter : DataTypeConversion  OutDataTypeStr=uint8
  convert_in : FVT_lib/hal/convert_in  gain=0.1  offset=0
  VHAL_PTC1PowerConsumption_kW : Outport
  wires:
  convert_in/1 -> VHAL_PTC1PowerConsumption_kW/1
  UnitConverter/1 -> convert_in/1
  PTC1_PowerConsumption/1 -> UnitConverter/1

== system halin/HAL_IN/CAN4/zGW_CANFr1/PTCActuPwrHSC6 ==
  PTCActuPwrHSC6 : Inport
  UnitConverter : DataTypeConversion  OutDataTypeStr=uint16
  VHAL_PTCActuPwrHSC6_enum : Outport
  wires:
  UnitConverter/1 -> VHAL_PTCActuPwrHSC6_enum/1
  PTCActuPwrHSC6/1 -> UnitConverter/1

== system halin/HAL_IN/CAN4/zGW_LINDr1/CSWDimSw ==
  CSW_DimSw : Inport
  UnitConverter : DataTypeConversion  OutDataTypeStr=uint8
  VHAL_CSWDimSw_flg : Outport
  wires:
  UnitConverter/1 -> VHAL_CSWDimSw_flg/1
  CSW_DimSw/1 -> UnitConverter/1

== system halin/HAL_IN/CAN4/zGW_LINDr1/CSWFWasSwSta ==
  CSW_FWasSw_Sta : Inport
  UnitConverter : DataTypeConversion  OutDataTypeStr=uint8
  VHAL_CSWFWasSwSta_enum : Outport
  wires:
  UnitConverter/1 -> VHAL_CSWFWasSwSta_enum/1
  CSW_FWasSw_Sta/1 -> UnitConverter/1

== system halin/HAL_IN/CAN4/zGW_LINDr1/CSWFWipSwSta ==
  CSW_FWipSw_Sta : Inport
  UnitConverter : DataTypeConversion  OutDataTypeStr=uint8
  VHAL_CSWFWipSwSta_enum : Outport
  wires:
  UnitConverter/1 -> VHAL_CSWFWipSwSta_enum/1
  CSW_FWipSw_Sta/1 -> UnitConverter/1

== system halin/HAL_IN/CAN4/zGW_LINDr1/CSWPassSWSta ==
  CSW_PassSW_Sta : Inport
  UnitConverter : DataTypeConversion  OutDataTypeStr=uint8
  VHAL_CSWPassSWSta_flg : Outport
  wires:
  UnitConverter/1 -> VHAL_CSWPassSWSta_flg/1
  CSW_PassSW_Sta/1 -> UnitConverter/1

== system halin/HAL_IN/CAN4/zGW_LINDr1/CSWRWasSWSta ==
  CSW_RWasSW_Sta : Inport
  UnitConverter : DataTypeConversion  OutDataTypeStr=uint8
  VHAL_CSWRWasSWSta_enum : Outport
  wires:
  UnitConverter/1 -> VHAL_CSWRWasSWSta_enum/1
  CSW_RWasSW_Sta/1 -> UnitConverter/1

== system halin/HAL_IN/CAN4/zGW_LINDr1/CSWRWipIntSwSta ==
  CSW_RWipIntSw_Sta : Inport
  UnitConverter : DataTypeConversion  OutDataTypeStr=uint8
  VHAL_CSWRWipIntSwSta_enum : Outport
  wires:
  UnitConverter/1 -> VHAL_CSWRWipIntSwSta_enum/1
  CSW_RWipIntSw_Sta/1 -> UnitConverter/1

== system halin/HAL_IN/CAN4/zGW_LINDr1/CSWTurnSwSta ==
  CSW_TurnSw_Sta : Inport
  UnitConverter : DataTypeConversion  OutDataTypeStr=uint8
  VHAL_CSWTurnSwSta_enum : Outport
  wires:
  UnitConverter/1 -> VHAL_CSWTurnSwSta_enum/1
  CSW_TurnSw_Sta/1 -> UnitConverter/1

== system halin/HAL_IN/CAN4/zGW_LINDr1/FAPWL01LINResponseError ==
  FAPWL_01_LIN_Response_Error : Inport
  UnitConverter : DataTypeConversion  OutDataTypeStr=uint8
  VHAL_FAPWL01LINResponseError_flg : Outport
  wires:
  UnitConverter/1 -> VHAL_FAPWL01LINResponseError_flg/1
  FAPWL_01_LIN_Response_Error/1 -> UnitConverter/1

== system halin/HAL_IN/CAN4/zGW_LINDr1/LDrvMotorRelayError ==
  L_Drv_Motor_Relay_Error : Inport
  UnitConverter : DataTypeConversion  OutDataTypeStr=uint8
  VHAL_LDrvMotorRelayError_flg : Outport
  wires:
  UnitConverter/1 -> VHAL_LDrvMotorRelayError_flg/1
  L_Drv_Motor_Relay_Error/1 -> UnitConverter/1

== system halin/HAL_IN/CAN4/zGW_LINDr1/LDrvMotorRippleError ==
  L_Drv_Motor_Ripple_Error : Inport
  UnitConverter : DataTypeConversion  OutDataTypeStr=uint8
  VHAL_LDrvMotorRippleError_flg : Outport
  wires:
  UnitConverter/1 -> VHAL_LDrvMotorRippleError_flg/1
  L_Drv_Motor_Ripple_Error/1 -> UnitConverter/1

== system halin/HAL_IN/CAN4/zGW_LINDr1/LDrvValWdwOpened ==
  L_Drv_Val_Wdw_Opened : Inport
  UnitConverter : DataTypeConversion  OutDataTypeStr=uint8
  VHAL_LDrvValWdwOpened_pct : Outport
  wires:
  UnitConverter/1 -> VHAL_LDrvValWdwOpened_pct/1
  L_Drv_Val_Wdw_Opened/1 -> UnitConverter/1

== system halin/HAL_IN/CAN4/zGW_LINDr1/LDrvWdwPositionSts ==
  L_Drv_Wdw_PositionSts : Inport
  UnitConverter : DataTypeConversion  OutDataTypeStr=uint8
  VHAL_LDrvWdwPositionSts_enum : Outport
  wires:
  UnitConverter/1 -> VHAL_LDrvWdwPositionSts_enum/1
  L_Drv_Wdw_PositionSts/1 -> UnitConverter/1

== system halin/HAL_IN/CAN4/zGW_LINDr1/LPasMotorRelayError ==
  L_Pas_Motor_Relay_Error : Inport
  UnitConverter : DataTypeConversion  OutDataTypeStr=uint8
  VHAL_LPasMotorRelayError_flg : Outport
  wires:
  UnitConverter/1 -> VHAL_LPasMotorRelayError_flg/1
  L_Pas_Motor_Relay_Error/1 -> UnitConverter/1

== system halin/HAL_IN/CAN4/zGW_LINDr1/LPasMotorRippleError ==
  L_Pas_Motor_Ripple_Error : Inport
  UnitConverter : DataTypeConversion  OutDataTypeStr=uint8
  VHAL_LPasMotorRippleError_flg : Outport
  wires:
  UnitConverter/1 -> VHAL_LPasMotorRippleError_flg/1
  L_Pas_Motor_Ripple_Error/1 -> UnitConverter/1

== system halin/HAL_IN/CAN4/zGW_LINDr1/LPasValWdwOpened ==
  L_Pas_Val_Wdw_Opened : Inport
  UnitConverter : DataTypeConversion  OutDataTypeStr=uint8
  VHAL_LPasValWdwOpened_pct : Outport
  wires:
  UnitConverter/1 -> VHAL_LPasValWdwOpened_pct/1
  L_Pas_Val_Wdw_Opened/1 -> UnitConverter/1

== system halin/HAL_IN/CAN4/zGW_LINDr1/LPasWdwPositionSts ==
  L_Pas_Wdw_PositionSts : Inport
  UnitConverter : DataTypeConversion  OutDataTypeStr=uint8
  VHAL_LPasWdwPositionSts_enum : Outport
  wires:
  UnitConverter/1 -> VHAL_LPasWdwPositionSts_enum/1
  L_Pas_Wdw_PositionSts/1 -> UnitConverter/1

== system halin/HAL_IN/CAN4/zGW_LINDr1/LRLDMotorRelayError ==
  L_RLD_Motor_Relay_Error : Inport
  UnitConverter : DataTypeConversion  OutDataTypeStr=uint8
  VHAL_LRLDMotorRelayError_flg : Outport
  wires:
  UnitConverter/1 -> VHAL_LRLDMotorRelayError_flg/1
  L_RLD_Motor_Relay_Error/1 -> UnitConverter/1

== system halin/HAL_IN/CAN4/zGW_LINDr1/LRLDMotorRippleError ==
  L_RLD_Motor_Ripple_Error : Inport
  UnitConverter : DataTypeConversion  OutDataTypeStr=uint8
  VHAL_LRLDMotorRippleError_flg : Outport
  wires:
  UnitConverter/1 -> VHAL_LRLDMotorRippleError_flg/1
  L_RLD_Motor_Ripple_Error/1 -> UnitConverter/1

== system halin/HAL_IN/CAN4/zGW_LINDr1/LRLDValWdwOpened ==
  L_RLD_Val_Wdw_Opened : Inport
  UnitConverter : DataTypeConversion  OutDataTypeStr=uint8
  VHAL_LRLDValWdwOpened_pct : Outport
  wires:
  UnitConverter/1 -> VHAL_LRLDValWdwOpened_pct/1
  L_RLD_Val_Wdw_Opened/1 -> UnitConverter/1

== system halin/HAL_IN/CAN4/zGW_LINDr1/LRLDWdwPositionSts ==
  L_RLD_Wdw_PositionSts : Inport
  UnitConverter : DataTypeConversion  OutDataTypeStr=uint8
  VHAL_LRLDWdwPositionSts_enum : Outport
  wires:
  UnitConverter/1 -> VHAL_LRLDWdwPositionSts_enum/1
  L_RLD_Wdw_PositionSts/1 -> UnitConverter/1

== system halin/HAL_IN/CAN4/zGW_LINDr1/LRRDMotorRelayError ==
  L_RRD_Motor_Relay_Error : Inport
  UnitConverter : DataTypeConversion  OutDataTypeStr=uint8
  VHAL_LRRDMotorRelayError_flg : Outport
  wires:
  UnitConverter/1 -> VHAL_LRRDMotorRelayError_flg/1
  L_RRD_Motor_Relay_Error/1 -> UnitConverter/1

== system halin/HAL_IN/CAN4/zGW_LINDr1/LRRDMotorRippleError ==
  L_RRD_Motor_Ripple_Error : Inport
  UnitConverter : DataTypeConversion  OutDataTypeStr=uint8
  VHAL_LRRDMotorRippleError_flg : Outport
  wires:
  UnitConverter/1 -> VHAL_LRRDMotorRippleError_flg/1
  L_RRD_Motor_Ripple_Error/1 -> UnitConverter/1

== system halin/HAL_IN/CAN4/zGW_LINDr1/LRRDValWdwOpened ==
  L_RRD_Val_Wdw_Opened : Inport
  UnitConverter : DataTypeConversion  OutDataTypeStr=uint8
  VHAL_LRRDValWdwOpened_pct : Outport
  wires:
  UnitConverter/1 -> VHAL_LRRDValWdwOpened_pct/1
  L_RRD_Val_Wdw_Opened/1 -> UnitConverter/1

== system halin/HAL_IN/CAN4/zGW_LINDr1/LRRDWdwPositionSts ==
  L_RRD_Wdw_PositionSts : Inport
  UnitConverter : DataTypeConversion  OutDataTypeStr=uint8
  VHAL_LRRDWdwPositionSts_enum : Outport
  wires:
  UnitConverter/1 -> VHAL_LRRDWdwPositionSts_enum/1
  L_RRD_Wdw_PositionSts/1 -> UnitConverter/1

== system halin/HAL_IN/CAN4/zGW_LINDr1/RAPWL01LINResponseError ==
  RAPWL_01_LIN_Response_Error : Inport
  UnitConverter : DataTypeConversion  OutDataTypeStr=uint8
  VHAL_RAPWL01LINResponseError_flg : Outport
  wires:
  UnitConverter/1 -> VHAL_RAPWL01LINResponseError_flg/1
  RAPWL_01_LIN_Response_Error/1 -> UnitConverter/1

== system halin/HAL_IN/CAN4/zGW_LINDr1/RLSLampSta ==
  RLS_Lamp_Sta : Inport
  UnitConverter : DataTypeConversion  OutDataTypeStr=uint8
  VHAL_RLSLampSta_flg : Outport
  wires:
  UnitConverter/1 -> VHAL_RLSLampSta_flg/1
  RLS_Lamp_Sta/1 -> UnitConverter/1

== system halin/HAL_IN/CAN4/zGW_LINDr1/RLSRainSnrWiperCmd ==
  RLS_RainSnrWiperCmd : Inport
  UnitConverter : DataTypeConversion  OutDataTypeStr=uint8
  VHAL_RLSRainSnrWiperCmd_enum : Outport
  wires:
  UnitConverter/1 -> VHAL_RLSRainSnrWiperCmd_enum/1
  RLS_RainSnrWiperCmd/1 -> UnitConverter/1

== system halin/HAL_IN/CAN4/zGW_LINDr1/SWC2LADASSta ==
  SWC2_L_ADAS_Sta : Inport
  UnitConverter : DataTypeConversion  OutDataTypeStr=uint8
  VHAL_SWC2LADASSta_flg : Outport
  wires:
  UnitConverter/1 -> VHAL_SWC2LADASSta_flg/1
  SWC2_L_ADAS_Sta/1 -> UnitConverter/1

== system halin/HAL_IN/CAN4/zGW_LINDr1/SWC2LDriveModeSta ==
  SWC2_L_DriveMode_Sta : Inport
  UnitConverter : DataTypeConversion  OutDataTypeStr=uint8
  VHAL_SWC2LDriveModeSta_flg : Outport
  wires:
  UnitConverter/1 -> VHAL_SWC2LDriveModeSta_flg/1
  SWC2_L_DriveMode_Sta/1 -> UnitConverter/1

== system halin/HAL_IN/CAN4/zGW_LINDr1/SWC2LHomeSta ==
  SWC2_L_Home_Sta : Inport
  UnitConverter : DataTypeConversion  OutDataTypeStr=uint8
  VHAL_SWC2LHomeSta_flg : Outport
  wires:
  UnitConverter/1 -> VHAL_SWC2LHomeSta_flg/1
  SWC2_L_Home_Sta/1 -> UnitConverter/1

== system halin/HAL_IN/CAN4/zGW_LINDr1/SWC2LLeftSta ==
  SWC2_L_Left_Sta : Inport
  UnitConverter : DataTypeConversion  OutDataTypeStr=uint8
  VHAL_SWC2LLeftSta_flg : Outport
  wires:
  UnitConverter/1 -> VHAL_SWC2LLeftSta_flg/1
  SWC2_L_Left_Sta/1 -> UnitConverter/1

== system halin/HAL_IN/CAN4/zGW_LINDr1/SWC2LRightSta ==
  SWC2_L_Right_Sta : Inport
  UnitConverter : DataTypeConversion  OutDataTypeStr=uint8
  VHAL_SWC2LRightSta_flg : Outport
  wires:
  UnitConverter/1 -> VHAL_SWC2LRightSta_flg/1
  SWC2_L_Right_Sta/1 -> UnitConverter/1

== system halin/HAL_IN/CAN4/zGW_LINDr1/SWC2LScrollDownSta ==
  SWC2_L_ScrollDown_Sta : Inport
  UnitConverter : DataTypeConversion  OutDataTypeStr=uint8
  VHAL_SWC2LScrollDownSta_flg : Outport
  wires:
  UnitConverter/1 -> VHAL_SWC2LScrollDownSta_flg/1
  SWC2_L_ScrollDown_Sta/1 -> UnitConverter/1

== system halin/HAL_IN/CAN4/zGW_LINDr1/SWC2LScrollPressSta ==
  SWC2_L_ScrollPress_Sta : Inport
  UnitConverter : DataTypeConversion  OutDataTypeStr=uint8
  VHAL_SWC2LScrollPressSta_flg : Outport
  wires:
  UnitConverter/1 -> VHAL_SWC2LScrollPressSta_flg/1
  SWC2_L_ScrollPress_Sta/1 -> UnitConverter/1

== system halin/HAL_IN/CAN4/zGW_LINDr1/SWC2LScrollUpSta ==
  SWC2_L_ScrollUp_Sta : Inport
  UnitConverter : DataTypeConversion  OutDataTypeStr=uint8
  VHAL_SWC2LScrollUpSta_flg : Outport
  wires:
  UnitConverter/1 -> VHAL_SWC2LScrollUpSta_flg/1
  SWC2_L_ScrollUp_Sta/1 -> UnitConverter/1

== system halin/HAL_IN/CAN4/zGW_LINDr1/SWC2RCustomizeSta ==
  SWC2_R_Customize_Sta : Inport
  UnitConverter : DataTypeConversion  OutDataTypeStr=uint8
  VHAL_SWC2RCustomizeSta_flg : Outport
  wires:
  UnitConverter/1 -> VHAL_SWC2RCustomizeSta_flg/1
  SWC2_R_Customize_Sta/1 -> UnitConverter/1

== system halin/HAL_IN/CAN4/zGW_LINDr1/SWC2RLeftSta ==
  SWC2_R_Left_Sta : Inport
  UnitConverter : DataTypeConversion  OutDataTypeStr=uint8
  VHAL_SWC2RLeftSta_flg : Outport
  wires:
  UnitConverter/1 -> VHAL_SWC2RLeftSta_flg/1
  SWC2_R_Left_Sta/1 -> UnitConverter/1

== system halin/HAL_IN/CAN4/zGW_LINDr1/SWC2RPageSwitchSta ==
  SWC2_R_PageSwitch_Sta : Inport
  UnitConverter : DataTypeConversion  OutDataTypeStr=uint8
  VHAL_SWC2RPageSwitchSta_flg : Outport
  wires:
  UnitConverter/1 -> VHAL_SWC2RPageSwitchSta_flg/1
  SWC2_R_PageSwitch_Sta/1 -> UnitConverter/1

== system halin/HAL_IN/CAN4/zGW_LINDr1/SWC2RRightSta ==
  SWC2_R_Right_Sta : Inport
  UnitConverter : DataTypeConversion  OutDataTypeStr=uint8
  VHAL_SWC2RRightSta_flg : Outport
  wires:
  UnitConverter/1 -> VHAL_SWC2RRightSta_flg/1
  SWC2_R_Right_Sta/1 -> UnitConverter/1

== system halin/HAL_IN/CAN4/zGW_LINDr1/SWC2RScrollDownSta ==
  SWC2_R_ScrollDown_Sta : Inport
  UnitConverter : DataTypeConversion  OutDataTypeStr=uint8
  VHAL_SWC2RScrollDownSta_flg : Outport
  wires:
  UnitConverter/1 -> VHAL_SWC2RScrollDownSta_flg/1
  SWC2_R_ScrollDown_Sta/1 -> UnitConverter/1

== system halin/HAL_IN/CAN4/zGW_LINDr1/SWC2RScrollPressSta ==
  SWC2_R_ScrollPress_Sta : Inport
  UnitConverter : DataTypeConversion  OutDataTypeStr=uint8
  VHAL_SWC2RScrollPressSta_flg : Outport
  wires:
  UnitConverter/1 -> VHAL_SWC2RScrollPressSta_flg/1
  SWC2_R_ScrollPress_Sta/1 -> UnitConverter/1

== system halin/HAL_IN/CAN4/zGW_LINDr1/SWC2RScrollUpSta ==
  SWC2_R_ScrollUp_Sta : Inport
  UnitConverter : DataTypeConversion  OutDataTypeStr=uint8
  VHAL_SWC2RScrollUpSta_flg : Outport
  wires:
  UnitConverter/1 -> VHAL_SWC2RScrollUpSta_flg/1
  SWC2_R_ScrollUp_Sta/1 -> UnitConverter/1

== system halin/HAL_IN/CAN4/zGW_LINDr1/SWC2RVRSta ==
  SWC2_R_VR_Sta : Inport
  UnitConverter : DataTypeConversion  OutDataTypeStr=uint8
  VHAL_SWC2RVRSta_flg : Outport
  wires:
  UnitConverter/1 -> VHAL_SWC2RVRSta_flg/1
  SWC2_R_VR_Sta/1 -> UnitConverter/1

== system halin/HAL_IN/CAN4/zGW_LINDr1/SWCACCSta ==
  SWC_ACC_Sta : Inport
  UnitConverter : DataTypeConversion  OutDataTypeStr=uint8
  VHAL_SWCACCSta_flg : Outport
  wires:
  UnitConverter/1 -> VHAL_SWCACCSta_flg/1
  SWC_ACC_Sta/1 -> UnitConverter/1

== system halin/HAL_IN/CAN4/zGW_LINDr1/SWCCANCELSta ==
  SWC_CANCEL_Sta : Inport
  UnitConverter : DataTypeConversion  OutDataTypeStr=uint8
  VHAL_SWCCANCELSta_flg : Outport
  wires:
  UnitConverter/1 -> VHAL_SWCCANCELSta_flg/1
  SWC_CANCEL_Sta/1 -> UnitConverter/1

== system halin/HAL_IN/CAN4/zGW_LINDr1/SWCDistanceSta ==
  SWC_Distance_Sta : Inport
  UnitConverter : DataTypeConversion  OutDataTypeStr=uint8
  VHAL_SWCDistanceSta_flg : Outport
  wires:
  UnitConverter/1 -> VHAL_SWCDistanceSta_flg/1
  SWC_Distance_Sta/1 -> UnitConverter/1

== system halin/HAL_IN/CAN4/zGW_LINDr1/SWCDownSta ==
  SWC_Down_Sta : Inport
  UnitConverter : DataTypeConversion  OutDataTypeStr=uint8
  VHAL_SWCDownSta_flg : Outport
  wires:
  UnitConverter/1 -> VHAL_SWCDownSta_flg/1
  SWC_Down_Sta/1 -> UnitConverter/1

== system halin/HAL_IN/CAN4/zGW_LINDr1/SWCLKASta ==
  SWC_LKA_Sta : Inport
  UnitConverter : DataTypeConversion  OutDataTypeStr=uint8
  VHAL_SWCLKASta_flg : Outport
  wires:
  UnitConverter/1 -> VHAL_SWCLKASta_flg/1
  SWC_LKA_Sta/1 -> UnitConverter/1

== system halin/HAL_IN/CAN4/zGW_LINDr1/SWCLeftSta ==
  SWC_Left_Sta : Inport
  UnitConverter : DataTypeConversion  OutDataTypeStr=uint8
  VHAL_SWCLeftSta_flg : Outport
  wires:
  UnitConverter/1 -> VHAL_SWCLeftSta_flg/1
  SWC_Left_Sta/1 -> UnitConverter/1

== system halin/HAL_IN/CAN4/zGW_LINDr1/SWCRegenDown ==
  SWC_RegenDown : Inport
  UnitConverter : DataTypeConversion  OutDataTypeStr=uint8
  VHAL_SWCRegenDown_flg : Outport
  wires:
  UnitConverter/1 -> VHAL_SWCRegenDown_flg/1
  SWC_RegenDown/1 -> UnitConverter/1

== system halin/HAL_IN/CAN4/zGW_LINDr1/SWCRegenUp ==
  SWC_RegenUp : Inport
  UnitConverter : DataTypeConversion  OutDataTypeStr=uint8
  VHAL_SWCRegenUp_flg : Outport
  wires:
  UnitConverter/1 -> VHAL_SWCRegenUp_flg/1
  SWC_RegenUp/1 -> UnitConverter/1

== system halin/HAL_IN/CAN4/zGW_LINDr1/SWCResUpSta ==
  SWC_Res_Up_Sta : Inport
  UnitConverter : DataTypeConversion  OutDataTypeStr=uint8
  VHAL_SWCResUpSta_flg : Outport
  wires:
  UnitConverter/1 -> VHAL_SWCResUpSta_flg/1
  SWC_Res_Up_Sta/1 -> UnitConverter/1

== system halin/HAL_IN/CAN4/zGW_LINDr1/SWCRightSta ==
  SWC_Right_Sta : Inport
  UnitConverter : DataTypeConversion  OutDataTypeStr=uint8
  VHAL_SWCRightSta_flg : Outport
  wires:
  UnitConverter/1 -> VHAL_SWCRightSta_flg/1
  SWC_Right_Sta/1 -> UnitConverter/1

== system halin/HAL_IN/CAN4/zGW_LINDr1/SWCSetdownSta ==
  SWC_Set_down_Sta : Inport
  UnitConverter : DataTypeConversion  OutDataTypeStr=uint8
  VHAL_SWCSetdownSta_flg : Outport
  wires:
  UnitConverter/1 -> VHAL_SWCSetdownSta_flg/1
  SWC_Set_down_Sta/1 -> UnitConverter/1

== system halin/HAL_IN/CAN4/zGW_LINDr1/SWCTripSta ==
  SWC_Trip_Sta : Inport
  UnitConverter : DataTypeConversion  OutDataTypeStr=uint8
  VHAL_SWCTripSta_flg : Outport
  wires:
  UnitConverter/1 -> VHAL_SWCTripSta_flg/1
  SWC_Trip_Sta/1 -> UnitConverter/1

== system halin/HAL_IN/CAN4/zGW_LINDr1/SWCUndefinedSta ==
  SWC_Undefined_Sta : Inport
  UnitConverter : DataTypeConversion  OutDataTypeStr=uint8
  VHAL_SWCUndefinedSta_flg : Outport
  wires:
  UnitConverter/1 -> VHAL_SWCUndefinedSta_flg/1
  SWC_Undefined_Sta/1 -> UnitConverter/1

== system halin/HAL_IN/CAN4/zGW_LINDr1/SWCUpSta ==
  SWC_Up_Sta : Inport
  UnitConverter : DataTypeConversion  OutDataTypeStr=uint8
  VHAL_SWCUpSta_flg : Outport
  wires:
  UnitConverter/1 -> VHAL_SWCUpSta_flg/1
  SWC_Up_Sta/1 -> UnitConverter/1

== system halin/HAL_IN/CAN4/zGW_LINDr1/SWCVRSta ==
  SWC_VR_Sta : Inport
  UnitConverter : DataTypeConversion  OutDataTypeStr=uint8
  VHAL_SWCVRSta_flg : Outport
  wires:
  UnitConverter/1 -> VHAL_SWCVRSta_flg/1
  SWC_VR_Sta/1 -> UnitConverter/1

== system halin/HAL_IN/CAN4/zGW_LINDr1/SWCmodeSta ==
  SWC_mode_Sta : Inport
  UnitConverter : DataTypeConversion  OutDataTypeStr=uint8
  VHAL_SWCmodeSta_flg : Outport
  wires:
  UnitConverter/1 -> VHAL_SWCmodeSta_flg/1
  SWC_mode_Sta/1 -> UnitConverter/1

== system halin/HAL_IN/CAN4/zGW_LINFr1/AGSActualPosition ==
  AGS_Actual_Position : Inport
  UnitConverter : DataTypeConversion  OutDataTypeStr=uint8
  VHAL_AGSActualPosition_enum : Outport
  wires:
  UnitConverter/1 -> VHAL_AGSActualPosition_enum/1
  AGS_Actual_Position/1 -> UnitConverter/1

== system halin/HAL_IN/CAN4/zGW_SEAT1/DSEATAntiSta ==
  DSEAT_Anti_Sta : Inport
  UnitConverter : DataTypeConversion  OutDataTypeStr=uint8
  VHAL_DSEATAntiSta_flg : Outport
  wires:
  UnitConverter/1 -> VHAL_DSEATAntiSta_flg/1
  DSEAT_Anti_Sta/1 -> UnitConverter/1

== system halin/HAL_IN/CAN4/zGW_SEAT1/DSEATEntryFunSta ==
  DSEAT_EntryFun_Sta : Inport
  UnitConverter : DataTypeConversion  OutDataTypeStr=uint8
  VHAL_DSEATEntryFunSta_flg : Outport
  wires:
  UnitConverter/1 -> VHAL_DSEATEntryFunSta_flg/1
  DSEAT_EntryFun_Sta/1 -> UnitConverter/1

== system halin/HAL_IN/CAN4/zGW_SEAT1/DSEATErrorSta ==
  DSEAT_Error_Sta : Inport
  UnitConverter : DataTypeConversion  OutDataTypeStr=uint8
  VHAL_DSEATErrorSta_flg : Outport
  wires:
  UnitConverter/1 -> VHAL_DSEATErrorSta_flg/1
  DSEAT_Error_Sta/1 -> UnitConverter/1

== system halin/HAL_IN/CAN4/zGW_SEAT1/DSEATHWVer ==
  DSEAT_HW_Ver : Inport
  UnitConverter : DataTypeConversion  OutDataTypeStr=uint16
  VHAL_DSEATHWVer_enum : Outport
  wires:
  UnitConverter/1 -> VHAL_DSEATHWVer_enum/1
  DSEAT_HW_Ver/1 -> UnitConverter/1

== system halin/HAL_IN/CAN4/zGW_SEAT1/DSEATMode ==
  DSEAT_Mode : Inport
  UnitConverter : DataTypeConversion  OutDataTypeStr=uint8
  VHAL_DSEATMode_enum : Outport
  wires:
  UnitConverter/1 -> VHAL_DSEATMode_enum/1
  DSEAT_Mode/1 -> UnitConverter/1

== system halin/HAL_IN/CAN4/zGW_SEAT1/DSEATSWVer ==
  DSEAT_SW_Ver : Inport
  UnitConverter : DataTypeConversion  OutDataTypeStr=uint16
  VHAL_DSEATSWVer_enum : Outport
  wires:
  UnitConverter/1 -> VHAL_DSEATSWVer_enum/1
  DSEAT_SW_Ver/1 -> UnitConverter/1

== system halin/HAL_IN/CAN4/zGW_SEAT1/DSEATVentSta ==
  DSEAT_Vent_Sta : Inport
  UnitConverter : DataTypeConversion  OutDataTypeStr=uint8
  VHAL_DSEATVentSta_enum : Outport
  wires:
  UnitConverter/1 -> VHAL_DSEATVentSta_enum/1
  DSEAT_Vent_Sta/1 -> UnitConverter/1

== system halin/HAL_IN/CAN4/zGW_SEAT1/DSEATheatersta ==
  DSEAT_heater_sta : Inport
  UnitConverter : DataTypeConversion  OutDataTypeStr=uint8
  VHAL_DSEATheatersta_enum : Outport
  wires:
  UnitConverter/1 -> VHAL_DSEATheatersta_enum/1
  DSEAT_heater_sta/1 -> UnitConverter/1

== system halin/HAL_IN/CAN4/zGW_SEAT1/PSEATErrorSta ==
  PSEAT_Error_Sta : Inport
  UnitConverter : DataTypeConversion  OutDataTypeStr=uint8
  VHAL_PSEATErrorSta_flg : Outport
  wires:
  UnitConverter/1 -> VHAL_PSEATErrorSta_flg/1
  PSEAT_Error_Sta/1 -> UnitConverter/1

== system halin/HAL_IN/CAN4/zGW_SEAT1/PSEATHWVer ==
  PSEAT_HW_Ver : Inport
  UnitConverter : DataTypeConversion  OutDataTypeStr=uint16
  VHAL_PSEATHWVer_enum : Outport
  wires:
  UnitConverter/1 -> VHAL_PSEATHWVer_enum/1
  PSEAT_HW_Ver/1 -> UnitConverter/1

== system halin/HAL_IN/CAN4/zGW_SEAT1/PSEATMode ==
  PSEAT_Mode : Inport
  UnitConverter : DataTypeConversion  OutDataTypeStr=uint8
  VHAL_PSEATMode_enum : Outport
  wires:
  UnitConverter/1 -> VHAL_PSEATMode_enum/1
  PSEAT_Mode/1 -> UnitConverter/1
